simulink model "Sender_Assignment_2"  (R2023b)
settings: Solver=FixedStepAuto  StartTime=0.0  StopTime=7.00  RelTol=1e-3
undefined symbols (not defined in the file): enable_decrypt, Key, Method, Seed, Sender_Final0x5B10x5D, SNR
libraries: androiduilib x5, androidsensorlib x2, androidaudiovideolib x1, androidcommunicationlib x1
settings Model: Creator=hp  LastModifiedBy=krish
settings OptimizationCC: EnhancedBackFolding=on  PassReuseOutputArgsThreshold=0  MaxStackSize=64  OptimizeBlockOrder=speed  DifferentSizesBufferReuse=on  OptimizationCustomize=off
settings DebuggingCC: ParameterTunabilityLossMsg=error
settings HardwareCC: ProdBitPerLong=64  ProdLargestAtomicInteger=LongLong  ProdLargestAtomicFloat=Double  ProdLongLongMode=on  ProdHWDeviceType=ARM Compatible->ARM Cortex-A (64-bit)  UseEmbeddedCoderFeatures=off  UseSimulinkCoderFeatures=off
settings SFSimCC: MATLABDynamicMemAlloc=off
settings RTWCC: Description=Embedded Coder  SystemTargetFile=ert.tlc  HardwareBoard=Android Device (64bit)  TLCOptions="-aInlineSetEventsForThisBaseRateFcn=TLC_FALSE -aSuppressMultiTaskScheduler=TLC_FALSE  -aRateBasedStepFcn=0"  TemplateMakefile=ert_default_tmf  RTWVerbose=off  Toolchain=Android SDK/NDK Tools
settings CodeAppCC: ForceParamTrailComments=on  OperatorAnnotations=on
settings ERTTargetCC: ERTCustomFileBanners=off  SupportContinuousTime=on  SupportNonInlinedSFcns=on  RemoveResetFunc=off  ModelStepFunctionPrototypeControlCompliant=off

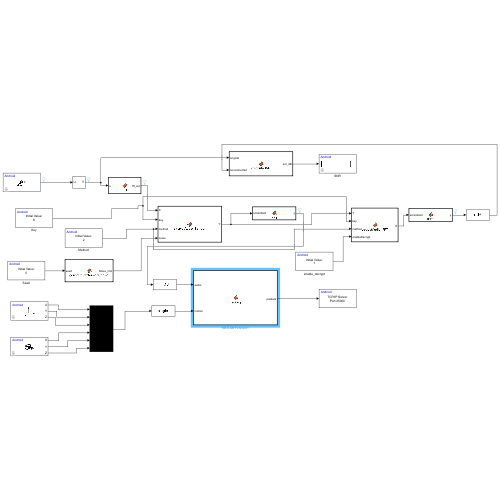
[thumbnail: Simulink's stored preview of the top-level diagram]
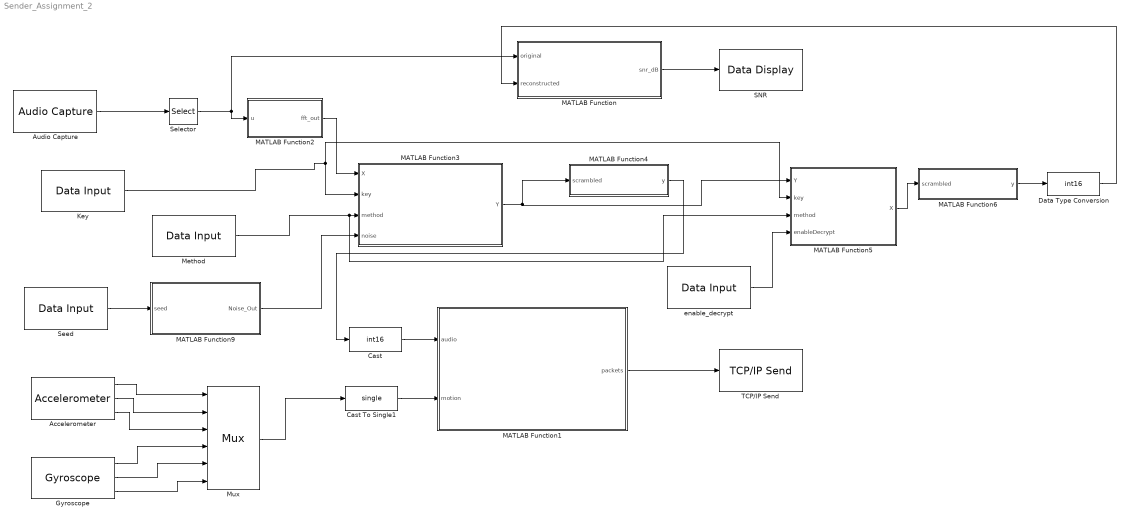
== system Sender_Assignment_2 ==
  Accelerometer : androidsensorlib/Accelerometer  OutputVector=off  SampleTime=0.1  BlockPlatform=Android
  Audio Capture : androidaudiovideolib/Audio Capture  SampleFreq=44100  FrameSize=4410  SampleTime=0.1  SimulateUsing=Code generation  DeviceStr=0  QueueDuration=0  BlockPlatform=Android  AudioSamplingFreq=44100
  Cast : DataTypeConversion  OutDataTypeStr=int16  SaturateOnIntegerOverflow=off  RndMeth=Floor
  Cast To Single1 : DataTypeConversion  OutDataTypeStr=single  SaturateOnIntegerOverflow=off  RndMeth=Floor
  Data Type Conversion : DataTypeConversion  OutDataTypeStr=int16  SaturateOnIntegerOverflow=off  RndMeth=Floor
  Gyroscope : androidsensorlib/Gyroscope  OutputVector=off  SampleTime=0.1  BlockPlatform=Android
  Key : androiduilib/Data Input  isCharVector=off  Value=6  CharVector=Hello World  OutputDataType=double  maxCharVectorSize=100  DataInputId=Sender_Final0x5B10x5D/Key  SampleTime=0.1
  MATLAB Function : MATLAB Function  TreatAsAtomicUnit=on
  MATLAB Function1 : MATLAB Function  TreatAsAtomicUnit=on
  MATLAB Function2 : MATLAB Function  TreatAsAtomicUnit=on
  MATLAB Function3 : MATLAB Function  TreatAsAtomicUnit=on
  MATLAB Function4 : MATLAB Function  TreatAsAtomicUnit=on
  MATLAB Function5 : MATLAB Function  TreatAsAtomicUnit=on
  MATLAB Function6 : MATLAB Function  TreatAsAtomicUnit=on
  MATLAB Function9 : MATLAB Function  TreatAsAtomicUnit=on
  Method : androiduilib/Data Input  isCharVector=off  Value=2  CharVector=Hello World  OutputDataType=double  maxCharVectorSize=100  DataInputId=Sender_Final0x5B10x5D/Method  SampleTime=0.1
  Mux : Mux  Inputs=6
  SNR : androiduilib/Data Display  DataDisplayId=Sender_Final0x5B10x5D/SNR  Format=Float  Precision=6  SimulateUsing=Code generation  blockPlatform=Android
  Seed : androiduilib/Data Input  isCharVector=off  Value=5  CharVector=Hello World  OutputDataType=double  maxCharVectorSize=100  DataInputId=Sender_Final0x5B10x5D/Seed  SampleTime=0.1
  Selector : Selector  NumberOfDimensions=2  InputPortWidth=3  IndexOptions=Select all,Index vector (dialog)  Indices=[1 3],1  OutputSizes=1,1
  TCP/IP Send : androidcommunicationlib/TCP//IP Send  TCPSendId=Sender_Final0x5B10x5D/TCP//IP_Send  Mode_=Server  LocalServerPort_=25000  RemoteAddr_=10.7.4.60  RemoteServerPort_=25000  ClientPortBindingSelection_=off  ClientPortToBind_=35000  BlockingMode_=on  BlockTimeout_=0.1
  enable_decrypt : androiduilib/Data Input  isCharVector=off  Value=1  CharVector=Hello World  OutputDataType=double  maxCharVectorSize=100  DataInputId=Sender_Final0x5B10x5D/enable_decrypt  SampleTime=0.1
  wires:
  Cast/1 -> MATLAB Function1/1(audio)
  Accelerometer/1 -> Mux/1
  Accelerometer/2 -> Mux/2
  Accelerometer/3 -> Mux/3
  Gyroscope/1 -> Mux/4
  Gyroscope/2 -> Mux/5
  Gyroscope/3 -> Mux/6
  Mux/1 -> Cast To Single1/1
  Cast To Single1/1 -> MATLAB Function1/2(motion)
  MATLAB Function4/1(y) -> Cast/1
  Selector/1 -> MATLAB Function/1(original), MATLAB Function2/1(u)
  MATLAB Function2/1(fft_out) -> MATLAB Function3/1(X)
  Key/1 -> MATLAB Function5/2(key), MATLAB Function3/2(key)
  Seed/1 -> MATLAB Function9/1(seed)
  MATLAB Function3/1(Y) -> MATLAB Function4/1(scrambled), MATLAB Function5/1(Y)
  MATLAB Function9/1(Noise_Out) -> MATLAB Function3/4(noise)
  Audio Capture/1 -> Selector/1
  MATLAB Function1/1(packets) -> TCP/IP Send/1
  MATLAB Function/1(snr_dB) -> SNR/1
  enable_decrypt/1 -> MATLAB Function5/4(enableDecrypt)
  MATLAB Function5/1(X) -> MATLAB Function6/1(scrambled)
  MATLAB Function6/1(y) -> Data Type Conversion/1
  Data Type Conversion/1 -> MATLAB Function/2(reconstructed)
  Method/1 -> MATLAB Function5/3(method), MATLAB Function3/3(method)

== matlab function Sender_Assignment_2/MATLAB Function1 ==
  data: audio input; packets output; motion input
function packets = packing(audio, motion)
assert(isa(motion,'single') && numel(motion)==6);
assert(isa(audio,'int16') && numel(audio)==4410);

packets = zeros(8844,1,'uint8');   % total = 24 + 8820

packets(1:24)    = typecast(motion(:), 'uint8').';        
packets(25:8844) = typecast(audio(:), 'uint8').';
end

== matlab function Sender_Assignment_2/MATLAB Function ==
  data: original input; snr_dB output; reconstructed input
function snr_dB = computeSNR(original, reconstructed)

    N = min(numel(original), numel(reconstructed));
    x = double(original(1:N));
    y = double(reconstructed(1:N));
    noise = x - y;

    Ps = mean(abs(x).^2);       % Signal Power
    Pn = mean(abs(noise).^2);   % Noise Power

    Ps = max(Ps, 1e-12);
    Pn = max(Pn, 1e-12);

    ratio = Ps / Pn;
    snr_dB = 10 * log10(ratio);
    snr_dB = real(snr_dB);
end

== matlab function Sender_Assignment_2/MATLAB Function5 ==
  data: Y input; X output; key input; method input; enableDecrypt input
function X = decryptAudio_FFT(Y, key, method, enableDecrypt)
    [N, C] = size(Y);
    X = complex(zeros(N, C, 'like', Y));
    
    if nargin < 4 || enableDecrypt == 0
        X = Y; return;
    end
    
    if ischar(key) || isstring(key)
        keyChar = double(char(key));
        keynum = sum(keyChar .* (1:length(keyChar))); 
    else
        keynum = double(key);
    end
    seedVal = max(1, floor(abs(keynum)));

    switch int16(method)
        
        % CASE 1: Unscramble
        case 1
            X = keyUnscrambleFFT(Y, seedVal);

        % CASE 2: Remove Adaptive Spectrum Noise
        case 2
            s = rng;
            rng(seedVal, 'twister');

            magY = abs(Y);
            magEnv = movmean(magY, 8, 1);

            noise_white = randn(N, C);
            f_bins = (1:N)';
            pink_filter = 1 ./ (sqrt(f_bins) + 1);
            noise_pink = noise_white .* pink_filter;

            normalized_env = magEnv ./ max(magEnv(:) + eps);
            noise_adaptive = noise_pink .* normalized_env;

            noise_level = 1000 * mean(magY(:)); 
            noise_final = noise_adaptive * noise_level;

            magRec = magY - abs(noise_final);
            magRec(magRec < 0) = 0;

            phaseY = angle(Y);
            X = magRec .* exp(1j * phaseY);

            rng(s);

            
        % CASE 3: Water Mark
        case 3
            X = Y; 
            
        otherwise
            X = Y;
    end
end

function X = keyUnscrambleFFT(Y, key)
    [N, C] = size(Y);
    posIdx = 2:floor(N/2);
    negIdx = N - posIdx + 2;
    K = numel(posIdx);
    if K == 0; X = Y; return; end
    b = mod(key, K); a = mod(key, K-1) + 1;
    while K > 1 && gcd(a, K) ~= 1; a = a + 1; if a >= K; a = 1; end; end
    [g, inv_a, ~] = gcd(a, K); inv_a = mod(inv_a, K);
    inv_perm = zeros(1, K);
    for m = 1:K; inv_perm(m) = mod(inv_a * ((m-1) - b), K) + 1; end
    if ~isreal(Y); X = complex(zeros(N, C, 'like', Y)); else; X = zeros(N, C, 'like', Y); end
    X(1, :) = Y(1, :);
    if mod(N,2) == 0; X(N/2 + 1, :) = Y(N/2 + 1, :); end
    X(posIdx, :) = Y(posIdx(inv_perm), :);
    if ~isreal(Y); X(negIdx, :) = conj(X(posIdx, :)); else; X(negIdx, :) = X(posIdx, :); end
end

== matlab function Sender_Assignment_2/MATLAB Function6 ==
  data: scrambled input; y output
function y = IFFT(scrambled)
    N = length(scrambled);
    scrambled(2:N/2) = conj(scrambled(N:-1:N/2+2));
    Channel = ifft(scrambled);
    y = real(Channel);
end

== matlab function Sender_Assignment_2/MATLAB Function2 ==
  data: u input; fft_out output
function fft_out = FFT(u)
    u = u(:,1);
    fft_out = fft(double(u));
end

== matlab function Sender_Assignment_2/MATLAB Function3 ==
  data: X input; Y output; key input; method input; noise input
function Y = encryptAudio_Sender(X, key, method, noise)
    [N, C] = size(X);
    
    if size(noise, 1) ~= N
        noise_safe = complex(zeros(N, C)); 
    else
        noise_safe = noise;
    end

    if ischar(key) || isstring(key)
        keyChar = double(char(key));
        keynum = sum(keyChar .* (1:length(keyChar))); 
    else
        keynum = double(key);
    end
    seedVal = max(1, floor(abs(keynum)));
    
    Y = complex(zeros(N, C, 'like', X));

    switch double(method)
        
        % METHOD 1: Frequency Scrambling (UNCHANGED)
        case 1 
            Y = keyScrambleFFT(X, seedVal);
            
        % METHOD 2: Adaptive Pink Noise Masking
        case 2 
            s = rng; 
            rng(seedVal, 'twister'); 
            
            magX = abs(X);
            magEnv = movmean(magX, 8, 1); 
            
            noise_white = randn(N, C);
            f_bins = (1:N)';
            pink_filter = 1 ./ (sqrt(f_bins) + 1);
            noise_pink = noise_white .* pink_filter;
            
            normalized_env = magEnv ./ max(magEnv(:) + eps);
            noise_adaptive = noise_pink .* normalized_env;
            
            noise_level = 1000 * mean(magX(:)); 
            noise_final = noise_adaptive * noise_level;
            
            phaseX = angle(X);
            magY = magX + abs(noise_final); 
            Y = magY .* exp(1j * phaseX);
            
            rng(s);

        % METHOD 3: Watermarking
        case 3
            Y = X + noise;
           
        otherwise
            Y = X;
    end
end

function Yout = keyScrambleFFT(Xin, key)
    [N, C] = size(Xin);
    posIdx = 2:floor(N/2);
    negIdx = N - posIdx + 2;
    K = numel(posIdx);
    if K == 0; Yout = Xin; return; end
    b = mod(key, K); a = mod(key, K-1) + 1;
    if K > 1; while gcd(a, K) ~= 1; a = a + 1; if a >= K; a = 1; end; end; end
    perm = zeros(1, K);
    for i = 0:(K-1); perm(i+1) = mod(a * i + b, K) + 1; end
    pidx = posIdx(perm);
    Yout = complex(zeros(N, C, 'like', Xin));
    Yout(1, :) = Xin(1, :);
    if mod(N, 2) == 0; Yout(N/2 + 1, :) = Xin(N/2 + 1, :); end
    Yout(posIdx, :) = Xin(pidx, :);
    Yout(negIdx, :) = conj(Yout(posIdx, :));
end

== matlab function Sender_Assignment_2/MATLAB Function4 ==
  data: scrambled input; y output
function y = IFFT(scrambled)
    N = length(scrambled);
    scrambled(2:N/2) = conj(scrambled(N:-1:N/2+2));
    Channel = ifft(scrambled);
    y = real(Channel);
end

== matlab function Sender_Assignment_2/MATLAB Function9 ==
  data: seed input; Noise_Out output
function Noise_Out = generate_watermark_noise(seed)
    % --- 1. Constants ---
    N = 4410; 
    Fs = 44100;
    df = Fs / N; % ~21.5 Hz per bin
    
    f_start_hz = 200;
    f_end_hz   = 15000;
    
    alpha = 5000; 

    % --- 2. Identify Target Bins ---
    idx_start = floor(f_start_hz / df) + 1;
    idx_end   = ceil(f_end_hz / df) + 1;
    
    % Clamp to Nyquist (Ensure we don't exceed 11025Hz)
    if idx_end > (N/2)
        idx_end = floor(N/2);
    end

    % --- 3. Generate Noise (Seed Dependent) ---
    rng(uint32(seed), 'twister');
    
    % Calculate bins to fill
    num_bins = idx_end - idx_start + 1;
    
    % Generate complex Gaussian noise
    noise_real = randn(num_bins, 1);
    noise_imag = randn(num_bins, 1);
    
    % Create the band noise
    noise_band = alpha * complex(noise_real, noise_imag);

    % --- 4. Assign to Output ---
    Noise_Out = complex(zeros(N, 1));
    
    % A. Positive Frequencies
    current_bin = 0;
    for i = idx_start : idx_end
        current_bin = current_bin + 1;
        Noise_Out(i) = noise_band(current_bin);
    end

    % B. Negative Frequencies (Conjugate Mirror)
    current_bin = 0;
    for k = idx_start : idx_end
        current_bin = current_bin + 1;
        mirror_idx = N - k + 2;
        
        if mirror_idx <= N
            Noise_Out(mirror_idx) = conj(noise_band(current_bin));
        end
    end

end
